simulink model "roverDynamics"  (R2021b)
settings: Solver=ode15s  StartTime=0  StopTime=20791  RelTol=1e-3
values from neighbouring files (symbols this model uses):
  beta = pi/2    (= 1.57079632679)    [compute_normal.m]    (also in initParams4Simulink.m; standardTerrainProfile.mat; standardTerrainProfile_long.mat; standardTerrainProfile_short.mat)
  g = -9.807    [compute_normal.m]    (also in initParams4Simulink.m; standardTerrainProfile.mat = -3.721; standardTerrainProfile_long.mat; standardTerrainProfile_short.mat)
  gamma = pi/2    (= 1.57079632679)    [compute_normal.m]    (also in initParams4Simulink.m; standardTerrainProfile.mat; standardTerrainProfile_long.mat; standardTerrainProfile_short.mat)
  l1 = 2    [compute_normal.m]    (also in initParams4Simulink.m; standardTerrainProfile.mat; standardTerrainProfile_long.mat; standardTerrainProfile_short.mat)
  l2 = 1    [compute_normal.m]    (also in initParams4Simulink.m; standardTerrainProfile.mat; standardTerrainProfile_long.mat; standardTerrainProfile_short.mat)
  l3 = 1    [compute_normal.m]    (also in initParams4Simulink.m; standardTerrainProfile.mat; standardTerrainProfile_long.mat; standardTerrainProfile_short.mat)
  lB = 1    [compute_normal.m]    (also in initParams4Simulink.m; standardTerrainProfile.mat; standardTerrainProfile_long.mat; standardTerrainProfile_short.mat)
  m = 10    [compute_normal.m]    (also in initParams4Simulink.m = 1025; init_rover.m = 100; standardTerrainProfile.mat = 1025; standardTerrainProfile_long.mat = 1025)
  phi_shift = 0.321750554397    [standardTerrainProfile.mat]    (also in workspace.mat)
  r = 0.25    [compute_normal.m]    (also in initParams4Simulink.m = 0.525; init_rover.m = 0.2; standardTerrainProfile.mat; standardTerrainProfile_long.mat = 0.525)
  theta1 = pi/2 - gamma/2    (= 0.785398163397)    [compute_normal.m]    (also in initParams4Simulink.m; standardTerrainProfile.mat; standardTerrainProfile_long.mat; standardTerrainProfile_short.mat)
  theta2 = pi/2 - beta/2    (= 0.785398163397)    [compute_normal.m]    (also in initParams4Simulink.m; standardTerrainProfile.mat; standardTerrainProfile_long.mat; standardTerrainProfile_short.mat)
  theta3 = pi/2 + beta/2    (= 2.35619449019)    [compute_normal.m]    (also in initParams4Simulink.m; standardTerrainProfile.mat = 0.785398163397; standardTerrainProfile_long.mat; standardTerrainProfile_short.mat)
  thetaB = pi/2 + gamma/2    (= 2.35619449019)    [compute_normal.m]    (also in initParams4Simulink.m; standardTerrainProfile.mat; standardTerrainProfile_long.mat; standardTerrainProfile_short.mat)
libraries: slpidlib x4
settings Model: Creator=matte  LastModifiedBy=matte

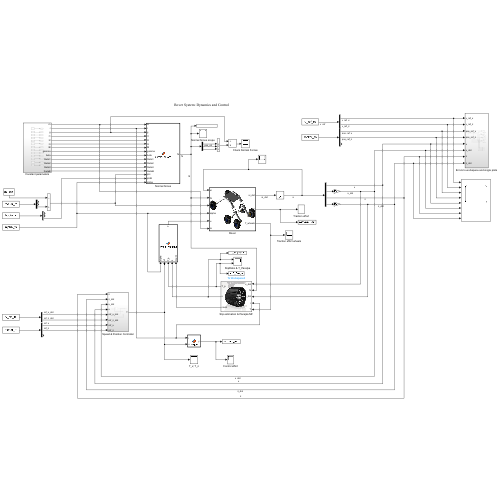
[thumbnail: Simulink's stored preview of the top-level diagram]
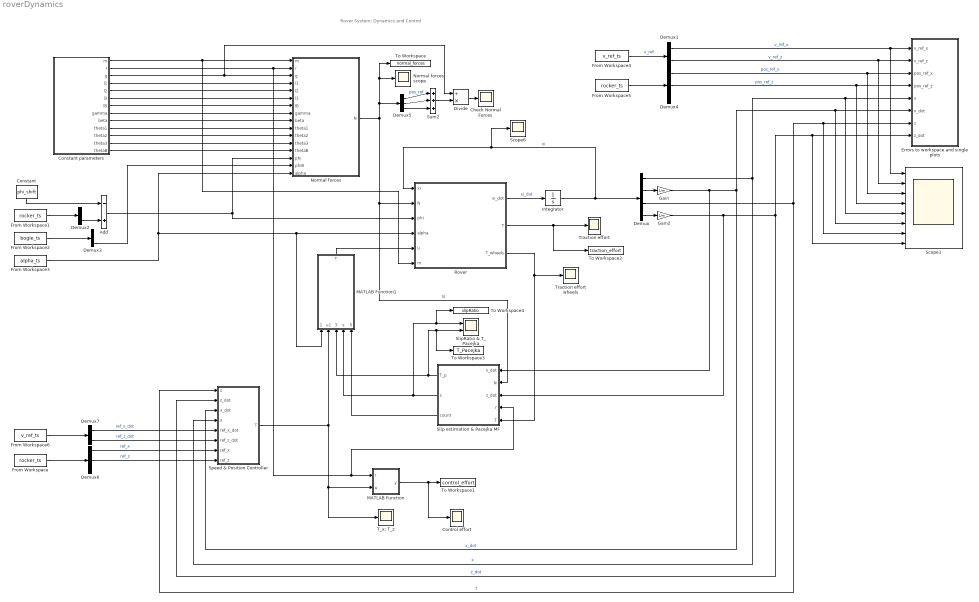
== system roverDynamics ==
  note: Rover System: Dynamics and Control
  Add : Sum  Inputs=-+
  Check Normal Forces : Scope
  Constant : Constant  Value=phi_shift
  Constant parameters : Subsystem
  Control effort : Scope
  Demux : Demux
  Demux1 : Demux  Outputs=2
  Demux{2..6} (5 alike) : Demux  Outputs=3
  Demux7 : Demux  Outputs=2
  Divide : Product  Inputs=/*
  Errors to workspace and single plots : Subsystem
  From Workspace : FromWorkspace  VariableName=rocker_ts
  From Workspace1 : FromWorkspace  VariableName=rocker_ts
  From Workspace2 : FromWorkspace  VariableName=bogie_ts
  From Workspace3 : FromWorkspace  VariableName=alpha_ts
  From Workspace4 : FromWorkspace  VariableName=v_ref_ts
  From Workspace5 : FromWorkspace  VariableName=rocker_ts
  From Workspace6 : FromWorkspace  VariableName=v_ref_ts
  Gain : Gain  Gain=1/m
  Gain2 : Gain  Gain=1/m
  Integrator : Integrator
  MATLAB Function : MATLAB Function  TreatAsAtomicUnit=on
  MATLAB Function1 : MATLAB Function  TreatAsAtomicUnit=on
  Normal forces : MATLAB Function  TreatAsAtomicUnit=on
  Normal forces scope : Scope
  Rover : MATLAB Function  TreatAsAtomicUnit=on
  Scope1 : Scope  NumInputPorts=8
  Scope6 : Scope
  Slip estimation & Pacejka MF : Subsystem
      mask Display: image('$imagefile'); % Use "Edit Image" on toolstrip to change.
  SlipRatio & T_Pacejka : Scope  NumInputPorts=2
  Speed & Position Controller : Subsystem
  Sum2 : Sum  Inputs=|+++
  T_x; T_z : Scope
  To Workspace : ToWorkspace  VariableName=normal_forces  SaveFormat=Timeseries  SampleTime=-1
  To Workspace1 : ToWorkspace  VariableName=control_effort  SaveFormat=Timeseries  SampleTime=-1
  To Workspace2 : ToWorkspace  VariableName=traction_effort  SaveFormat=Timeseries  SampleTime=-1
  To Workspace3 : ToWorkspace  VariableName=T_Pacejka  SaveFormat=Timeseries  SampleTime=-1
  To Workspace4 : ToWorkspace  VariableName=slipRatio  SaveFormat=Timeseries  SampleTime=-1
  Traction effort : Scope
  Traction effort wheels : Scope
  wires:
  From Workspace5/1 -> Demux4/1
  Constant/1 -> Add/1
  Constant parameters/8(gamma) -> Normal forces/8(gamma)
  Constant parameters/9(beta) -> Normal forces/9(beta)
  Add/1 -> Normal forces/14(phi), Rover/3(phi)
  Constant parameters/5(l2) -> Normal forces/5(l2)
  Rover/1(xi_dot) -> Integrator/1  "xi_dot"
  Constant parameters/3(g) -> Divide/1, Normal forces/3(g)
  Divide/1 -> Check Normal Forces/1
  Demux5/3 -> Sum2/3
  Demux5/1 -> Sum2/1  "pos_ref"
  Demux5/2 -> Sum2/2
  Constant parameters/13(thetaB) -> Normal forces/13(thetaB)
  Sum2/1 -> Divide/2
  Constant parameters/7(lB) -> Normal forces/7(lB)
  Constant parameters/12(theta3) -> Normal forces/12(theta3)
  Demux/1 -> Speed & Position Controller/4(x), Scope1/5, Errors to workspace and single plots/5(x)  "x"
  Constant parameters/4(l1) -> Normal forces/4(l1)
  Constant parameters/6(l3) -> Normal forces/6(l3)
  From Workspace1/1 -> Demux2/1
  Constant parameters/11(theta2) -> Normal forces/11(theta2)
  Constant parameters/1(m) -> Rover/6(m), Normal forces/1(m)
  Demux2/3 -> Add/2
  Demux/2 -> Gain/1
  From Workspace2/1 -> Demux3/1
  Demux3/3 -> Normal forces/15(phiB)
  Normal forces/1(N) -> Demux5/1, Normal forces scope/1, To Workspace/1, Rover/2(N), Slip estimation & Pacejka MF/2(N)  "N"
  From Workspace3/1 -> Normal forces/16(alpha), MATLAB Function1/1(alpha), Rover/4(alpha)
  Constant parameters/10(theta1) -> Normal forces/10(theta1)
  Integrator/1 -> Demux/1, Scope6/1, Rover/1(xi)  "xi"
  From Workspace/1 -> Demux6/1
  Gain2/1 -> Slip estimation & Pacejka MF/3(z_dot), Speed & Position Controller/2(z_dot), Scope1/8, Errors to workspace and single plots/8(z_dot)  "z_dot"
  Demux/3 -> Speed & Position Controller/1(z), Scope1/7, Errors to workspace and single plots/7(z)  "z"
  Demux/4 -> Gain2/1
  From Workspace6/1 -> Demux7/1
  MATLAB Function/1(y) -> Control effort/1, To Workspace1/1
  Demux6/1 -> Speed & Position Controller/7(ref_x)  "ref_x"
  Demux6/2 -> Speed & Position Controller/8(ref_z)  "ref_z"
  Gain/1 -> Slip estimation & Pacejka MF/1(x_dot), Speed & Position Controller/3(x_dot), Scope1/6, Errors to workspace and single plots/6(x_dot)  "x_dot"
  From Workspace4/1 -> Demux1/1  "v_ref"
  Demux1/1 -> Scope1/1, Errors to workspace and single plots/1(v_ref_x)  "v_ref_x"
  Demux1/2 -> Scope1/2, Errors to workspace and single plots/2(v_ref_z)  "v_ref_z"
  Demux4/1 -> Scope1/3, Errors to workspace and single plots/3(pos_ref_x)  "pos_ref_x"
  Demux4/2 -> Scope1/4, Errors to workspace and single plots/4(pos_ref_z)  "pos_ref_z"
  MATLAB Function1/1(T) -> Rover/5(u)
  Demux7/1 -> Speed & Position Controller/5(ref_x_dot)  "ref_x_dot"
  Demux7/2 -> Speed & Position Controller/6(ref_z_dot)  "ref_z_dot"
  Speed & Position Controller/1(T) -> MATLAB Function1/2(u1), MATLAB Function/2(u), T_x; T_z/1
  Rover/2(T) -> To Workspace2/1, Traction effort/1
  Rover/3(T_wheels) -> Slip estimation & Pacejka MF/5(T), Traction effort wheels/1
  Slip estimation & Pacejka MF/1(T_p) -> To Workspace3/1, SlipRatio & T_Pacejka/2, MATLAB Function1/3(T_p)
  Slip estimation & Pacejka MF/2(s) -> To Workspace4/1, SlipRatio & T_Pacejka/1, MATLAB Function1/4(s)
  Slip estimation & Pacejka MF/3(count) -> MATLAB Function1/5(count)
  Constant parameters/2(r) -> Normal forces/2(r), Slip estimation & Pacejka MF/4(r), MATLAB Function/1(r)

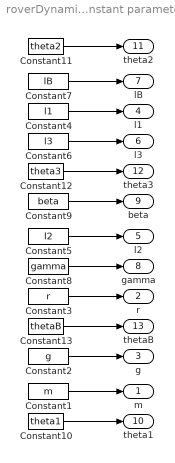
== system roverDynamics/Constant parameters ==
  Constant1 : Constant  Value=m
  Constant10 : Constant  Value=theta1
  Constant11 : Constant  Value=theta2
  Constant12 : Constant  Value=theta3
  Constant13 : Constant  Value=thetaB
  Constant2 : Constant  Value=g
  Constant3 : Constant  Value=r
  Constant4 : Constant  Value=l1
  Constant5 : Constant  Value=l2
  Constant6 : Constant  Value=l3
  Constant7 : Constant  Value=lB
  Constant8 : Constant  Value=gamma
  Constant9 : Constant  Value=beta
  m : Outport
  r : Outport  Port=2
  g : Outport  Port=3
  l1 : Outport  Port=4
  l2 : Outport  Port=5
  l3 : Outport  Port=6
  lB : Outport  Port=7
  gamma : Outport  Port=8
  beta : Outport  Port=9
  theta1 : Outport  Port=10
  theta2 : Outport  Port=11
  theta3 : Outport  Port=12
  thetaB : Outport  Port=13
  wires:
  Constant6/1 -> l3/1
  Constant2/1 -> g/1
  Constant9/1 -> beta/1
  Constant5/1 -> l2/1
  Constant11/1 -> theta2/1
  Constant7/1 -> lB/1
  Constant4/1 -> l1/1
  Constant12/1 -> theta3/1
  Constant13/1 -> thetaB/1
  Constant3/1 -> r/1
  Constant10/1 -> theta1/1
  Constant8/1 -> gamma/1
  Constant1/1 -> m/1

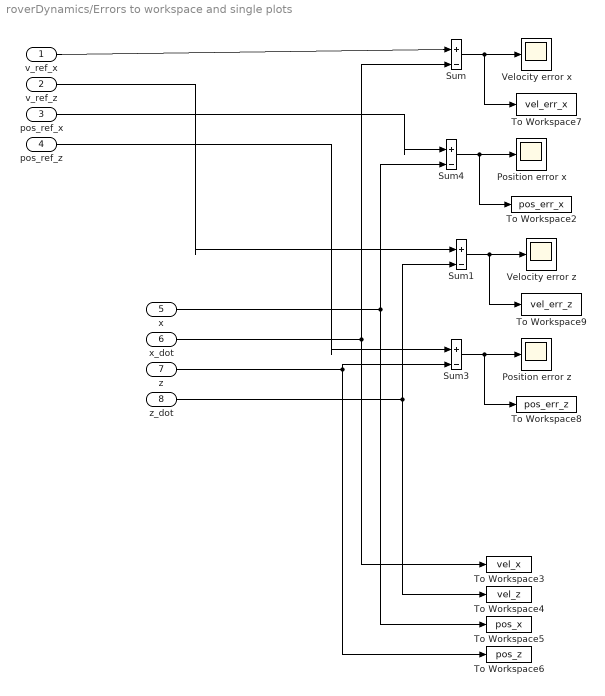
== system roverDynamics/Errors to workspace and single plots ==
  v_ref_x : Inport
  v_ref_z : Inport  Port=2
  pos_ref_x : Inport  Port=3
  pos_ref_z : Inport  Port=4
  x : Inport  Port=5
  x_dot : Inport  Port=6
  z : Inport  Port=7
  z_dot : Inport  Port=8
  Position error x : Scope
  Position error z : Scope
  Sum{,1,3..4} (4 alike) : Sum  Inputs=|+-
  To Workspace2 : ToWorkspace  VariableName=pos_err_x  SaveFormat=Timeseries  SampleTime=-1
  To Workspace3 : ToWorkspace  VariableName=vel_x  SaveFormat=Timeseries  SampleTime=-1
  To Workspace4 : ToWorkspace  VariableName=vel_z  SaveFormat=Timeseries  SampleTime=-1
  To Workspace5 : ToWorkspace  VariableName=pos_x  SaveFormat=Timeseries  SampleTime=-1
  To Workspace6 : ToWorkspace  VariableName=pos_z  SaveFormat=Timeseries  SampleTime=-1
  To Workspace7 : ToWorkspace  VariableName=vel_err_x  SaveFormat=Timeseries  SampleTime=-1
  To Workspace8 : ToWorkspace  VariableName=pos_err_z  SaveFormat=Timeseries  SampleTime=-1
  To Workspace9 : ToWorkspace  VariableName=vel_err_z  SaveFormat=Timeseries  SampleTime=-1
  Velocity error x : Scope
  Velocity error z : Scope
  wires:
  Sum3/1 -> To Workspace8/1, Position error z/1
  x_dot/1 -> Sum/2, To Workspace3/1
  x/1 -> To Workspace5/1, Sum4/2
  Sum/1 -> To Workspace7/1, Velocity error x/1
  Sum1/1 -> To Workspace9/1, Velocity error z/1
  v_ref_x/1 -> Sum/1
  Sum4/1 -> To Workspace2/1, Position error x/1
  pos_ref_x/1 -> Sum4/1
  z/1 -> Sum3/2, To Workspace6/1
  z_dot/1 -> To Workspace4/1, Sum1/2
  v_ref_z/1 -> Sum1/1
  pos_ref_z/1 -> Sum3/1

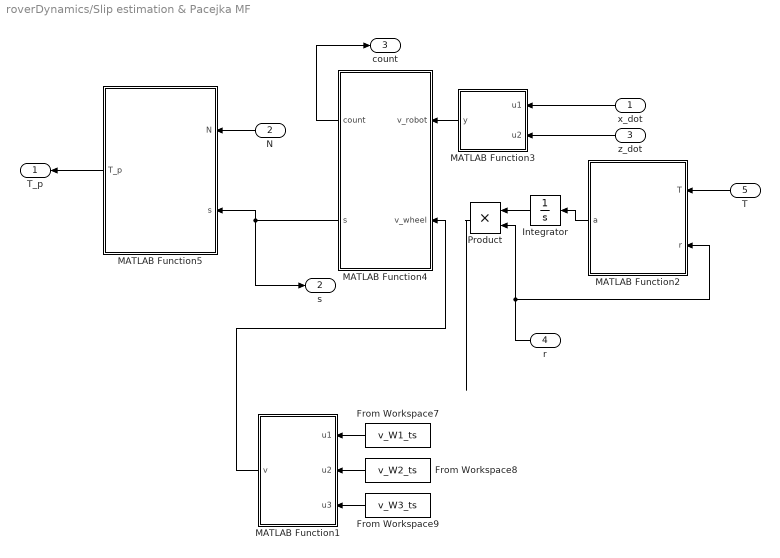
== system roverDynamics/Slip estimation & Pacejka MF ==
  x_dot : Inport
  N : Inport  Port=2
  z_dot : Inport  Port=3
  r : Inport  Port=4
  T : Inport  Port=5
  From Workspace7 : FromWorkspace  VariableName=v_W1_ts
  From Workspace8 : FromWorkspace  VariableName=v_W2_ts
  From Workspace9 : FromWorkspace  VariableName=v_W3_ts
  Integrator : Integrator
  MATLAB Function1 : MATLAB Function  TreatAsAtomicUnit=on
  MATLAB Function2 : MATLAB Function  TreatAsAtomicUnit=on
  MATLAB Function3 : MATLAB Function  TreatAsAtomicUnit=on
  MATLAB Function4 : MATLAB Function  TreatAsAtomicUnit=on
  MATLAB Function5 : MATLAB Function  TreatAsAtomicUnit=on
  Product : Product
  T_p : Outport
  s : Outport  Port=2
  count : Outport  Port=3
  wires:
  MATLAB Function4/2(s) -> MATLAB Function5/2(s), s/1
  From Workspace9/1 -> MATLAB Function1/3(u3)
  MATLAB Function3/1(y) -> MATLAB Function4/1(v_robot)
  x_dot/1 -> MATLAB Function3/1(u1)
  From Workspace8/1 -> MATLAB Function1/2(u2)
  N/1 -> MATLAB Function5/1(N)
  z_dot/1 -> MATLAB Function3/2(u2)
  MATLAB Function4/1(count) -> count/1
  From Workspace7/1 -> MATLAB Function1/1(u1)
  MATLAB Function5/1(T_p) -> T_p/1
  MATLAB Function2/1(a) -> Integrator/1
  Integrator/1 -> Product/1
  Product/1 -> ?
  r/1 -> MATLAB Function2/2(r), Product/2
  T/1 -> MATLAB Function2/1(T)
  MATLAB Function1/1(v) -> MATLAB Function4/2(v_wheel)

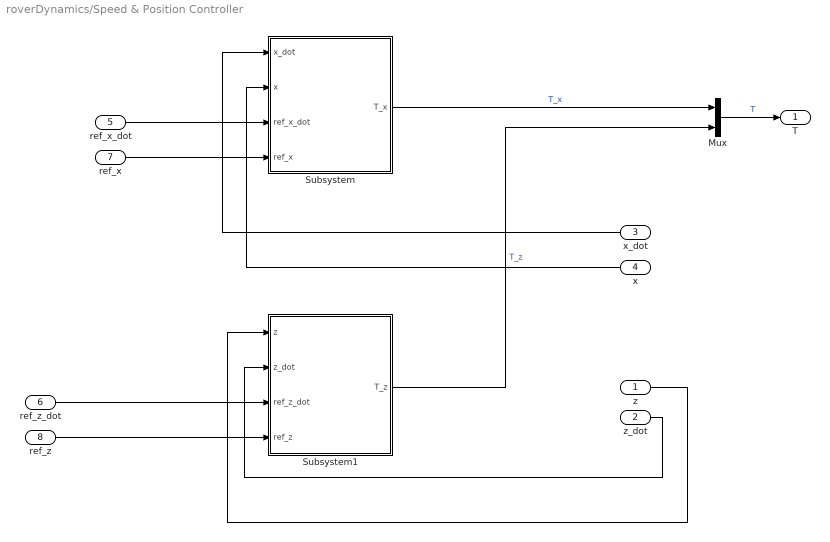
== system roverDynamics/Speed & Position Controller ==
  z : Inport
  z_dot : Inport  Port=2
  x_dot : Inport  Port=3
  x : Inport  Port=4
  ref_x_dot : Inport  Port=5
  ref_z_dot : Inport  Port=6
  ref_x : Inport  Port=7
  ref_z : Inport  Port=8
  Mux : Mux  Inputs=2
  Subsystem : Subsystem
  Subsystem1 : Subsystem
  T : Outport
  wires:
  x_dot/1 -> Subsystem/1(x_dot)
  Subsystem/1(T_x) -> Mux/1  "T_x"
  ref_x_dot/1 -> Subsystem/3(ref_x_dot)
  ref_z/1 -> Subsystem1/4(ref_z)
  Subsystem1/1(T_z) -> Mux/2  "T_z"
  ref_z_dot/1 -> Subsystem1/3(ref_z_dot)
  Mux/1 -> T/1  "T"
  ref_x/1 -> Subsystem/4(ref_x)
  x/1 -> Subsystem/2(x)
  z_dot/1 -> Subsystem1/2(z_dot)
  z/1 -> Subsystem1/1(z)

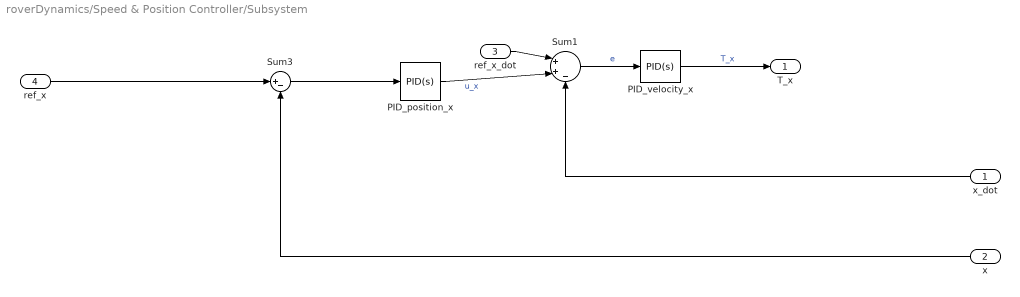
== system roverDynamics/Speed & Position Controller/Subsystem ==
  x_dot : Inport
  x : Inport  Port=2
  ref_x_dot : Inport  Port=3
  ref_x : Inport  Port=4
  PID_position_x : slpidlib/PID Controller  Controller=PID  Form=Parallel  TimeDomain=Continuous-time  UseExternalTs=off  SampleTime=-1  IntegratorMethod=Forward Euler  FilterMethod=Forward Euler  ControllerParametersSource=internal  P=19.9029545148168  I=35.1881636907475  D=1.75883934758459  UseFilter=on  N=191.088758350368  TunerSelectOption=Transfer Function Based (PID Tuner App)  InitialConditionSource=internal  InitialConditionForIntegrator=0  InitialConditionForFilter=0  DifferentiatorICPrevScaledInput=0  ExternalReset=none  TrackingMode=off  Kt=1  LimitOutput=off  SatLimitsSource=internal  UpperSaturationLimit=inf  LowerSaturationLimit=-inf  LinearizeAsGain=on  AntiWindupMode=none  Kb=1  POutMin=[]  POutMax=[]  IOutMin=[]  IOutMax=[]  DOutMin=[]  DOutMax=[]  NOutMin=[]  NOutMax=[]  SumOutMin=[]  SumOutMax=[]  SaturationOutMin=[]  SaturationOutMax=[]  PParamMin=[]  PParamMax=[]  IParamMin=[]  IParamMax=[]  DParamMin=[]  DParamMax=[]  NParamMin=[]  NParamMax=[]  KbParamMin=[]  KbParamMax=[]  KtParamMin=[]  KtParamMax=[]  KbOutMin=[]  KbOutMax=[]  KtOutMin=[]  KtOutMax=[]  IntegratorOutMin=[]  IntegratorOutMax=[]  FilterOutMin=[]  FilterOutMax=[]  SumI1OutMin=[]  SumI1OutMax=[]  SumI2OutMin=[]  SumI2OutMax=[]  SumI3OutMin=[]  SumI3OutMax=[]  SumI4OutMin=[]  SumI4OutMax=[]  SumDOutMin=[]  SumDOutMax=[]  DifferentiatorOutMin=[]  DifferentiatorOutMax=[]  FilterDiffOutCoefMin=[]  FilterDiffOutCoefMax=[]  ReciprocalOutMin=[]  ReciprocalOutMax=[]  SumDenOutMin=[]  SumDenOutMax=[]  SumNumOutMin=[]  SumNumOutMax=[]  DivideOutMin=[]  DivideOutMax=[]  UdiffTsProdOutMin=[]  UdiffTsProdOutMax=[]  NTsProdOutMin=[]  NTsProdOutMax=[]  UintegralTsProdOutMin=[]  UintegralTsProdOutMax=[]  UngainTsProdOutMin=[]  UngainTsProdOutMax=[]  IntegratorContinuousStateAttributes=''  IntegratorStateMustResolveToSignalObject=off  IntegratorRTWStateStorageClass=Auto  FilterContinuousStateAttributes=''  FilterStateMustResolveToSignalObject=off  FilterRTWStateStorageClass=Auto  ParallelPVariant=InternalParameters  IdealPVariant=Disabled  IVariant=InternalParameters  DVariant=InternalParameters  IntegratorVariant=Continuous  SatVariant=Disabled  AWVariant=Passthrough  PCopyVariant=Disabled  TRVariant=Disabled  FdbkBlocksVariant=Forward  IdealPFdbkVariant=Disabled  SatFdbkVariant=Disabled  DerivativeFilterVariant=ContFilter  NVariant=InternalParameters  NCopyVariant=Disabled  FilterICVariant=InternalICsFilter  IntegratorICVariant=InternalICs  ExternalResetVariant=Disabled  TRSumVariant=Passthrough  SumFdbkVariant=Disabled  SumVariant=Sum_PID  TsampFilterVariant=InternalTs  TsampNgainVariant=Passthrough  TsampIntegralVariant=Passthrough  ExternalSaturationOutDataTypeStr=Inherit: Same as second input
  PID_velocity_x : slpidlib/PID Controller  Controller=PID  Form=Parallel  TimeDomain=Continuous-time  UseExternalTs=off  SampleTime=-1  IntegratorMethod=Forward Euler  FilterMethod=Forward Euler  ControllerParametersSource=internal  P=4888.24294038826  I=8634.11342932201  D=92.833278012426  UseFilter=on  N=36.46824066771  TunerSelectOption=Transfer Function Based (PID Tuner App)  InitialConditionSource=internal  InitialConditionForIntegrator=0  InitialConditionForFilter=0  DifferentiatorICPrevScaledInput=0  ExternalReset=none  TrackingMode=off  Kt=1  LimitOutput=off  SatLimitsSource=internal  UpperSaturationLimit=inf  LowerSaturationLimit=-inf  LinearizeAsGain=on  AntiWindupMode=none  Kb=1  POutMin=[]  POutMax=[]  IOutMin=[]  IOutMax=[]  DOutMin=[]  DOutMax=[]  NOutMin=[]  NOutMax=[]  SumOutMin=[]  SumOutMax=[]  SaturationOutMin=[]  SaturationOutMax=[]  PParamMin=[]  PParamMax=[]  IParamMin=[]  IParamMax=[]  DParamMin=[]  DParamMax=[]  NParamMin=[]  NParamMax=[]  KbParamMin=[]  KbParamMax=[]  KtParamMin=[]  KtParamMax=[]  KbOutMin=[]  KbOutMax=[]  KtOutMin=[]  KtOutMax=[]  IntegratorOutMin=[]  IntegratorOutMax=[]  FilterOutMin=[]  FilterOutMax=[]  SumI1OutMin=[]  SumI1OutMax=[]  SumI2OutMin=[]  SumI2OutMax=[]  SumI3OutMin=[]  SumI3OutMax=[]  SumI4OutMin=[]  SumI4OutMax=[]  SumDOutMin=[]  SumDOutMax=[]  DifferentiatorOutMin=[]  DifferentiatorOutMax=[]  FilterDiffOutCoefMin=[]  FilterDiffOutCoefMax=[]  ReciprocalOutMin=[]  ReciprocalOutMax=[]  SumDenOutMin=[]  SumDenOutMax=[]  SumNumOutMin=[]  SumNumOutMax=[]  DivideOutMin=[]  DivideOutMax=[]  UdiffTsProdOutMin=[]  UdiffTsProdOutMax=[]  NTsProdOutMin=[]  NTsProdOutMax=[]  UintegralTsProdOutMin=[]  UintegralTsProdOutMax=[]  UngainTsProdOutMin=[]  UngainTsProdOutMax=[]  IntegratorContinuousStateAttributes=''  IntegratorStateMustResolveToSignalObject=off  IntegratorRTWStateStorageClass=Auto  FilterContinuousStateAttributes=''  FilterStateMustResolveToSignalObject=off  FilterRTWStateStorageClass=Auto  ParallelPVariant=InternalParameters  IdealPVariant=Disabled  IVariant=InternalParameters  DVariant=InternalParameters  IntegratorVariant=Continuous  SatVariant=Disabled  AWVariant=Passthrough  PCopyVariant=Disabled  TRVariant=Disabled  FdbkBlocksVariant=Forward  IdealPFdbkVariant=Disabled  SatFdbkVariant=Disabled  DerivativeFilterVariant=ContFilter  NVariant=InternalParameters  NCopyVariant=Disabled  FilterICVariant=InternalICsFilter  IntegratorICVariant=InternalICs  ExternalResetVariant=Disabled  TRSumVariant=Passthrough  SumFdbkVariant=Disabled  SumVariant=Sum_PID  TsampFilterVariant=InternalTs  TsampNgainVariant=Passthrough  TsampIntegralVariant=Passthrough  ExternalSaturationOutDataTypeStr=Inherit: Same as second input
  Sum1 : Sum  Inputs=|++-
  Sum3 : Sum  Inputs=|+-
  T_x : Outport
  wires:
  PID_position_x/1 -> Sum1/2  "u_x"
  PID_velocity_x/1 -> T_x/1  "T_x"
  ref_x_dot/1 -> Sum1/1
  x_dot/1 -> Sum1/3
  Sum3/1 -> PID_position_x/1
  x/1 -> Sum3/2
  ref_x/1 -> Sum3/1
  Sum1/1 -> PID_velocity_x/1  "e"

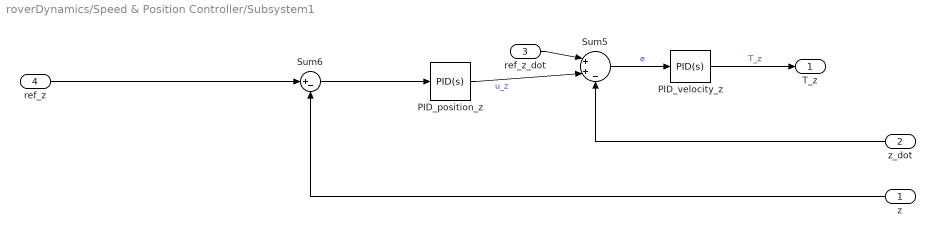
== system roverDynamics/Speed & Position Controller/Subsystem1 ==
  z : Inport
  z_dot : Inport  Port=2
  ref_z_dot : Inport  Port=3
  ref_z : Inport  Port=4
  PID_position_z : slpidlib/PID Controller  Controller=PID  Form=Parallel  TimeDomain=Continuous-time  UseExternalTs=off  SampleTime=-1  IntegratorMethod=Forward Euler  FilterMethod=Forward Euler  ControllerParametersSource=internal  P=18.6793914475963  I=33.1025727603455  D=1.70626396571439  UseFilter=on  N=182.488347496608  TunerSelectOption=Transfer Function Based (PID Tuner App)  InitialConditionSource=internal  InitialConditionForIntegrator=0  InitialConditionForFilter=0  DifferentiatorICPrevScaledInput=0  ExternalReset=none  TrackingMode=off  Kt=1  LimitOutput=off  SatLimitsSource=internal  UpperSaturationLimit=inf  LowerSaturationLimit=-inf  LinearizeAsGain=on  AntiWindupMode=none  Kb=1  POutMin=[]  POutMax=[]  IOutMin=[]  IOutMax=[]  DOutMin=[]  DOutMax=[]  NOutMin=[]  NOutMax=[]  SumOutMin=[]  SumOutMax=[]  SaturationOutMin=[]  SaturationOutMax=[]  PParamMin=[]  PParamMax=[]  IParamMin=[]  IParamMax=[]  DParamMin=[]  DParamMax=[]  NParamMin=[]  NParamMax=[]  KbParamMin=[]  KbParamMax=[]  KtParamMin=[]  KtParamMax=[]  KbOutMin=[]  KbOutMax=[]  KtOutMin=[]  KtOutMax=[]  IntegratorOutMin=[]  IntegratorOutMax=[]  FilterOutMin=[]  FilterOutMax=[]  SumI1OutMin=[]  SumI1OutMax=[]  SumI2OutMin=[]  SumI2OutMax=[]  SumI3OutMin=[]  SumI3OutMax=[]  SumI4OutMin=[]  SumI4OutMax=[]  SumDOutMin=[]  SumDOutMax=[]  DifferentiatorOutMin=[]  DifferentiatorOutMax=[]  FilterDiffOutCoefMin=[]  FilterDiffOutCoefMax=[]  ReciprocalOutMin=[]  ReciprocalOutMax=[]  SumDenOutMin=[]  SumDenOutMax=[]  SumNumOutMin=[]  SumNumOutMax=[]  DivideOutMin=[]  DivideOutMax=[]  UdiffTsProdOutMin=[]  UdiffTsProdOutMax=[]  NTsProdOutMin=[]  NTsProdOutMax=[]  UintegralTsProdOutMin=[]  UintegralTsProdOutMax=[]  UngainTsProdOutMin=[]  UngainTsProdOutMax=[]  IntegratorContinuousStateAttributes=''  IntegratorStateMustResolveToSignalObject=off  IntegratorRTWStateStorageClass=Auto  FilterContinuousStateAttributes=''  FilterStateMustResolveToSignalObject=off  FilterRTWStateStorageClass=Auto  ParallelPVariant=InternalParameters  IdealPVariant=Disabled  IVariant=InternalParameters  DVariant=InternalParameters  IntegratorVariant=Continuous  SatVariant=Disabled  AWVariant=Passthrough  PCopyVariant=Disabled  TRVariant=Disabled  FdbkBlocksVariant=Forward  IdealPFdbkVariant=Disabled  SatFdbkVariant=Disabled  DerivativeFilterVariant=ContFilter  NVariant=InternalParameters  NCopyVariant=Disabled  FilterICVariant=InternalICsFilter  IntegratorICVariant=InternalICs  ExternalResetVariant=Disabled  TRSumVariant=Passthrough  SumFdbkVariant=Disabled  SumVariant=Sum_PID  TsampFilterVariant=InternalTs  TsampNgainVariant=Passthrough  TsampIntegralVariant=Passthrough  ExternalSaturationOutDataTypeStr=Inherit: Same as second input
  PID_velocity_z : slpidlib/PID Controller  Controller=PID  Form=Parallel  TimeDomain=Continuous-time  UseExternalTs=off  SampleTime=-1  IntegratorMethod=Forward Euler  FilterMethod=Forward Euler  ControllerParametersSource=internal  P=4888.24294043909  I=8634.1134294118  D=92.8332780133915  UseFilter=on  N=36.46824066771  TunerSelectOption=Transfer Function Based (PID Tuner App)  InitialConditionSource=internal  InitialConditionForIntegrator=0  InitialConditionForFilter=0  DifferentiatorICPrevScaledInput=0  ExternalReset=none  TrackingMode=off  Kt=1  LimitOutput=off  SatLimitsSource=internal  UpperSaturationLimit=inf  LowerSaturationLimit=-inf  LinearizeAsGain=on  AntiWindupMode=none  Kb=1  POutMin=[]  POutMax=[]  IOutMin=[]  IOutMax=[]  DOutMin=[]  DOutMax=[]  NOutMin=[]  NOutMax=[]  SumOutMin=[]  SumOutMax=[]  SaturationOutMin=[]  SaturationOutMax=[]  PParamMin=[]  PParamMax=[]  IParamMin=[]  IParamMax=[]  DParamMin=[]  DParamMax=[]  NParamMin=[]  NParamMax=[]  KbParamMin=[]  KbParamMax=[]  KtParamMin=[]  KtParamMax=[]  KbOutMin=[]  KbOutMax=[]  KtOutMin=[]  KtOutMax=[]  IntegratorOutMin=[]  IntegratorOutMax=[]  FilterOutMin=[]  FilterOutMax=[]  SumI1OutMin=[]  SumI1OutMax=[]  SumI2OutMin=[]  SumI2OutMax=[]  SumI3OutMin=[]  SumI3OutMax=[]  SumI4OutMin=[]  SumI4OutMax=[]  SumDOutMin=[]  SumDOutMax=[]  DifferentiatorOutMin=[]  DifferentiatorOutMax=[]  FilterDiffOutCoefMin=[]  FilterDiffOutCoefMax=[]  ReciprocalOutMin=[]  ReciprocalOutMax=[]  SumDenOutMin=[]  SumDenOutMax=[]  SumNumOutMin=[]  SumNumOutMax=[]  DivideOutMin=[]  DivideOutMax=[]  UdiffTsProdOutMin=[]  UdiffTsProdOutMax=[]  NTsProdOutMin=[]  NTsProdOutMax=[]  UintegralTsProdOutMin=[]  UintegralTsProdOutMax=[]  UngainTsProdOutMin=[]  UngainTsProdOutMax=[]  IntegratorContinuousStateAttributes=''  IntegratorStateMustResolveToSignalObject=off  IntegratorRTWStateStorageClass=Auto  FilterContinuousStateAttributes=''  FilterStateMustResolveToSignalObject=off  FilterRTWStateStorageClass=Auto  ParallelPVariant=InternalParameters  IdealPVariant=Disabled  IVariant=InternalParameters  DVariant=InternalParameters  IntegratorVariant=Continuous  SatVariant=Disabled  AWVariant=Passthrough  PCopyVariant=Disabled  TRVariant=Disabled  FdbkBlocksVariant=Forward  IdealPFdbkVariant=Disabled  SatFdbkVariant=Disabled  DerivativeFilterVariant=ContFilter  NVariant=InternalParameters  NCopyVariant=Disabled  FilterICVariant=InternalICsFilter  IntegratorICVariant=InternalICs  ExternalResetVariant=Disabled  TRSumVariant=Passthrough  SumFdbkVariant=Disabled  SumVariant=Sum_PID  TsampFilterVariant=InternalTs  TsampNgainVariant=Passthrough  TsampIntegralVariant=Passthrough  ExternalSaturationOutDataTypeStr=Inherit: Same as second input
  Sum5 : Sum  Inputs=|++-
  Sum6 : Sum  Inputs=|+-
  T_z : Outport
  wires:
  z/1 -> Sum6/2
  PID_position_z/1 -> Sum5/2  "u_z"
  Sum6/1 -> PID_position_z/1
  Sum5/1 -> PID_velocity_z/1  "e"
  ref_z/1 -> Sum6/1
  PID_velocity_z/1 -> T_z/1  "T_z"
  z_dot/1 -> Sum5/3
  ref_z_dot/1 -> Sum5/1

== matlab function roverDynamics/Slip estimation & Pacejka MF/MATLAB Function4 ==
  data: count output; v_robot input; s output size=[3,1]; v_wheel input
function [count,s] = slipEstimator(v_robot,v_wheel)

if v_wheel(1) >= v_robot
    s1 = (v_wheel(1)-v_robot)/v_wheel(1); % accelerating
else
    s1 = (v_wheel(1)-v_robot)/v_robot; % decelerating
end

if v_wheel(2) >= v_robot
    s2 = (v_wheel(2)-v_robot)/v_wheel(2); % accelerating
else
    s2 = (v_wheel(2)-v_robot)/v_robot; % decelerating
end

if v_wheel(3) >= v_robot
    s3 = (v_wheel(3)-v_robot)/v_wheel(3); % accelerating
else
    s3 = (v_wheel(3)-v_robot)/v_robot; % decelerating
end

s = [s1,s2,s3]';

count = 0;

for i = 1:length(s)
    if abs(s(i))>0.9
        count = count+1;
    end
end

== matlab function roverDynamics/Slip estimation & Pacejka MF/MATLAB Function5 ==
  data: N input; s input; T_p output

function T_p = pacejkaMagicFormula(N,s)

surface = 3; % Surface choice : 1 - Dry Tarmac, 2 - Wet Tarmac, 3 - Snow, 4 - Ice
mu = zeros(1,3);
T_p = zeros(1,3);
B_tot = [10,12,5,4];
C_tot = [1.9,2.3,2,2];
D_tot = [1,0.82,0.3,0.1];
E_tot = [0.97,1,1,1];

B = B_tot(surface);
C = C_tot(surface);
D = D_tot(surface);
E = E_tot(surface);

for i = 1:length(s)
    mu(i) = D*sin(C*atan(B*s(i)-E*(B*s(i)-atan(B*s(i)))));
    T_p(i) = mu(i)*(-N(i));
end

== matlab function roverDynamics/Slip estimation & Pacejka MF/MATLAB Function1 ==
  data: u1 input; v output; u2 input; u3 input
function v = wheelVelocities(u1,u2,u3)
v1 = norm(u1(1),u1(2));
v2 = norm(u2(2),u2(2));
v3 = norm(u3(1),u3(2));

v = [v1;v2;v3];

== matlab function roverDynamics/Rover ==
  data: xi_dot output size=4; T output; T_wheels output size=3; xi input size=4; N input size=3; phi input size=1; alpha input size=3; u input size=6; m input
function [xi_dot, T,T_wheels]  = dyn(xi, N, phi, alpha, u, m)

c1 = cos(alpha(1));
c2 = cos(alpha(2));
c3 = cos(alpha(3));
s1 = sin(alpha(1));
s2 = sin(alpha(2));
s3 = sin(alpha(3));

T = u;

%% X & Z coordinates 

A = [0 1/m 0 0; 0 0 0 0; 0 0 0 1/m; 0 0 0 0];

B = [0 0 0 0 0 0; 1 1 1 0 0 0; 0 0 0 0 0 0; 0 0 0 1 1 1];

PSI = [0 0 0; s1 s2 s3; 0 0 0; c1 c2 c3]*N;

xi_dot = A*xi + B*T + PSI;

T1 = norm(u(1),u(4));
T2 = norm(u(2),u(5));
T3 = norm(u(3),u(6));

T_wheels = [T1;T2;T3];

== matlab function roverDynamics/MATLAB Function ==
  data: r input; u input; y output
function y = torque(r,u)

y = norm(u)*r;

== matlab function roverDynamics/MATLAB Function1 ==
  data: alpha input; u1 input; T output; T_p input; s input; count input
function T = wheelTractions(alpha,u1,T_p,s,count)

c1 = cos(alpha(1));
c2 = cos(alpha(2));
c3 = cos(alpha(3));
s1 = sin(alpha(1));
s2 = sin(alpha(2));
s3 = sin(alpha(3));

slipThreashold = 0.7;

T_tot = u1;
T_start = 1/3*T_tot;

Tx = [T_start(1);T_start(1);T_start(1)];
Tz = [T_start(2);T_start(2);T_start(2)];

T = [Tx;Tz];

pacejkaMode = 0;

if pacejkaMode == 1
    for i = 1: length(T_p)
        %if abs(mod(T(i),T(i+length(T_p))))>T_p(i)
        %if abs(s(i))>0.9
            %if count == 3
            T(i) = cos(alpha(i))*T_p(i);
            T(i+length(T_p)) = sin(alpha(i))*T_p(i);
        %end
    end
end

== matlab function roverDynamics/Normal forces ==
  data: m input; r input; g input; l1 input; l2 input; l3 input; lB input; gamma input; beta input; theta1 input; theta2 input; theta3 input; thetaB input; phi input; N output size=3; phiB input size=1; alpha input size=3
function N = normal_forces(m,r,g,l1,l2,l3,lB,gamma,beta,theta1,theta2,theta3, thetaB, phi, phiB, alpha)

%% ground to pivot vectors
R = [cos(phi) -sin(phi); sin(phi) cos(phi)];
RB = [cos(phiB) -sin(phiB); sin(phiB) cos(phiB)];

a = R*[l1*cos(theta1)-r*sin(alpha(1)); l1*sin(theta1)+r*cos(alpha(1))];
b = R*[lB*cos(thetaB); lB*sin(thetaB)];
c = R*RB*[l2*cos(theta2)-r*sin(alpha(2)); l2*sin(theta2)+r*cos(alpha(2))];
d = R*RB*[l3*cos(theta3)-r*sin(alpha(3)); l3*sin(theta3)+r*cos(alpha(3))];

% a = [l1*cos(theta1)-r*sin(alpha(1)); l1*sin(theta1)+r*cos(alpha(1))];
% b = [lB*cos(thetaB); lB*sin(thetaB)];
% c = RB*[l2*cos(theta2)-r*sin(alpha(2)); l2*sin(theta2)+r*cos(alpha(2))];
% d = RB*[l3*cos(theta3)-r*sin(alpha(3)); l3*sin(theta3)+r*cos(alpha(3))];

w = a-b;
e = RB*[-sin(alpha(1)), cos(alpha(1)); -cos(alpha(1)), -sin(alpha(1))]*w;

a_ = abs(a(1));
b_ = abs(b(1));
c_ = abs(c(1));
d_ = abs(d(1));

%% Forces
F = m*g;
F1 = F*(b_/(a_+b_));
FB = F*(a_/(a_+b_));
F2 = FB*(d_/(c_+d_));
F3 = FB*(c_/(c_+d_));

N = [F1; F2; F3];

end

== matlab function roverDynamics/Slip estimation & Pacejka MF/MATLAB Function2 ==
  data: T input; a output; r input
function a = wheelAngularAcc(T,r)
m = 2.75; % mass of a wheel
I = 0.5*m*(r^2);
a = zeros(3,1);

for i=1:length(T)
    a(i) = (r*T(i))/I;
end

== matlab function roverDynamics/Slip estimation & Pacejka MF/MATLAB Function3 ==
  data: u1 input; y output; u2 input
function y = norm(u1,u2)

y = norm(u1,u2);
